simulink model "sm_obs_dis"  (R2023b)
settings: Solver=VariableStepAuto  StartTime=0.0  StopTime=25.0  RelTol=1e-3
undefined symbols (not defined in the file): A_dis, B_dis, C_dis, k_dis, L_dis, tm
settings Model: Creator=yonathan  LastModifiedBy=yonathan

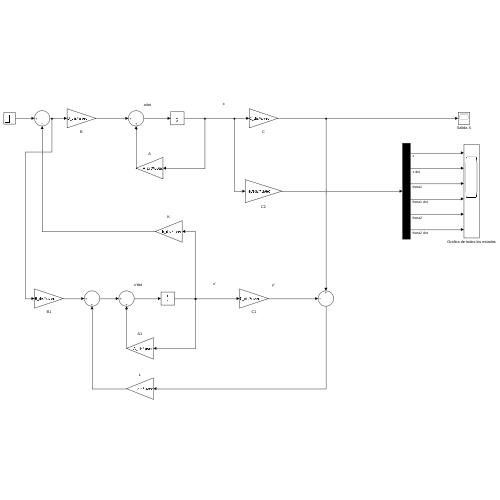
[thumbnail: Simulink's stored preview of the top-level diagram]
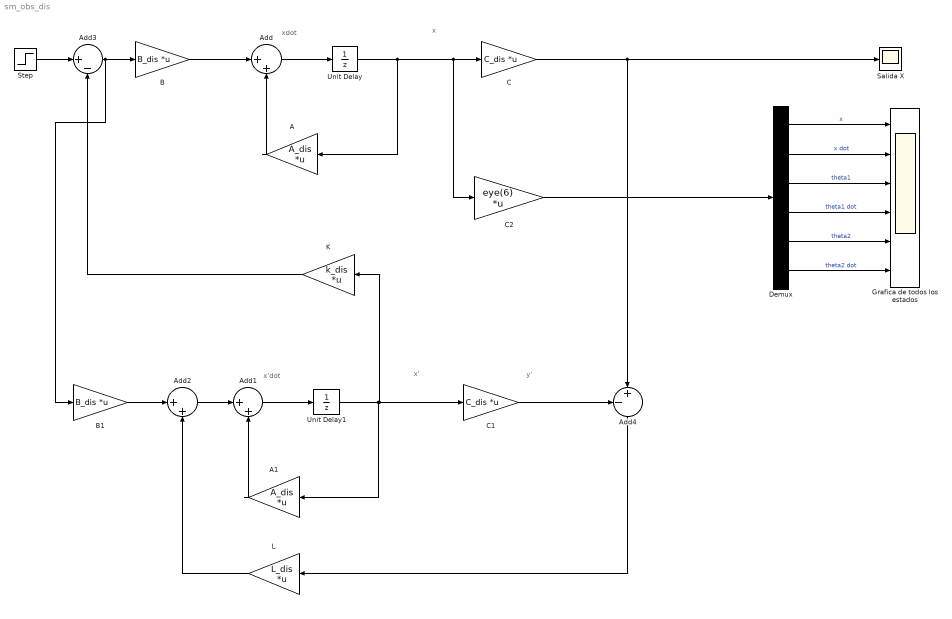
== system sm_obs_dis ==
  note: y'
  note: x
  note: xdot
  note: x'dot
  note: x'
  A : Gain  Gain=A_dis  Multiplication=Matrix(K*u) (u vector)
  A1 : Gain  Gain=A_dis  Multiplication=Matrix(K*u) (u vector)
  Add : Sum  Inputs=|++
  Add1 : Sum  Inputs=|++
  Add2 : Sum  Inputs=|++
  Add3 : Sum  Inputs=|+-
  Add4 : Sum  Inputs=-+|
  B : Gain  Gain=B_dis  Multiplication=Matrix(K*u) (u vector)
  B1 : Gain  Gain=B_dis  Multiplication=Matrix(K*u) (u vector)
  C : Gain  Gain=C_dis  Multiplication=Matrix(K*u) (u vector)
  C1 : Gain  Gain=C_dis  Multiplication=Matrix(K*u) (u vector)
  C2 : Gain  Gain=eye(6)  Multiplication=Matrix(K*u) (u vector)
  Demux : Demux  Outputs=6
  Grafica de todos los estados : Scope  NumInputPorts=6
  K : Gain  Gain=k_dis  Multiplication=Matrix(K*u) (u vector)
  L : Gain  Gain=L_dis  Multiplication=Matrix(K*u) (u vector)
  Salida X : Scope
  Step : Step  SampleTime=0
  Unit Delay : UnitDelay  SampleTime=tm  HasFrameUpgradeWarning=on
  Unit Delay1 : UnitDelay  SampleTime=tm  HasFrameUpgradeWarning=on
  wires:
  B/1 -> Add/1
  Unit Delay/1 -> A/1, C/1, C2/1
  A/1 -> Add/2
  C/1 -> Add4/2, Salida X/1
  Add/1 -> Unit Delay/1
  Add3/1 -> B1/1, B/1
  Add1/1 -> Unit Delay1/1
  A1/1 -> Add1/2
  Unit Delay1/1 -> A1/1, K/1, C1/1
  Add2/1 -> Add1/1
  B1/1 -> Add2/1
  Step/1 -> Add3/1
  K/1 -> Add3/2
  L/1 -> Add2/2
  C1/1 -> Add4/1
  Add4/1 -> L/1
  C2/1 -> Demux/1
  Demux/6 -> Grafica de todos los estados/6  "theta2 dot"
  Demux/5 -> Grafica de todos los estados/5  "theta2"
  Demux/4 -> Grafica de todos los estados/4  "theta1 dot"
  Demux/3 -> Grafica de todos los estados/3  "theta1"
  Demux/2 -> Grafica de todos los estados/2  "x dot"
  Demux/1 -> Grafica de todos los estados/1  "x"
